simulink subsystem "Day1_Scenario_1"  (R2024a)
settings: Solver=VariableStepAuto  StartTime=0.0  StopTime=10.0  RelTol=1e-3
libraries: CarMaker4SL x1
settings Model: Creator=junhyung.cha  LastModifiedBy=User

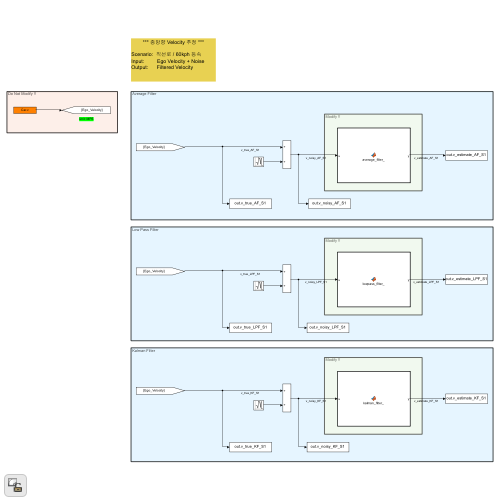
[thumbnail: Simulink's stored preview of the top-level diagram]
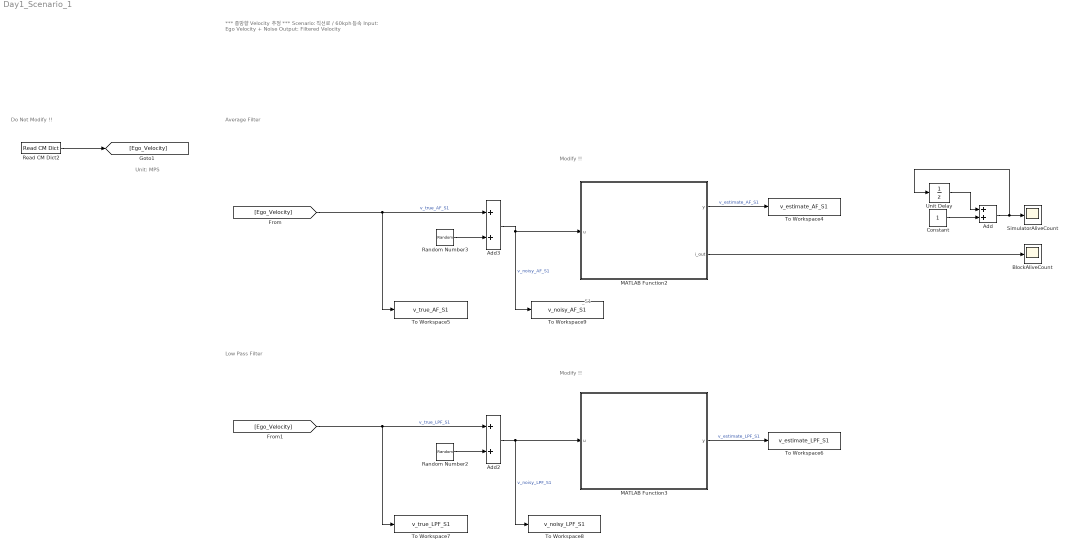
== system Day1_Scenario_1 ==
  note: _S1
  note: Modify !!
  note: Modify !!
  note: Average Filter
  note: Low Pass Filter
  note: *** 종방향 Velocity 추정 ***
      |
      | Scenario: 직선로 / 60kph 등속
      | Input: Ego Velocity + Noise
      | Output: Filtered Velocity
  note: Do Not Modify !!
  note: Unit: MPS
  Add : Sum
  Add2 : Sum
  Add3 : Sum
  BlockAliveCount : Scope
  Constant : Constant  SampleTime=-1
  MATLAB Function2 : MATLAB Function  TreatAsAtomicUnit=on
  MATLAB Function3 : MATLAB Function  TreatAsAtomicUnit=on
  Random Number2 : RandomNumber
  Random Number3 : RandomNumber
  Read CM Dict2 : CarMaker4SL/Read CM Dict  xname=Car.v  xsync=off  xstime=Inherited
  SimulatorAliveCount : Scope
  To Workspace4 : ToWorkspace  VariableName=v_estimate_AF_S1  SaveFormat=Timeseries  SampleTime=-1
  To Workspace5 : ToWorkspace  VariableName=v_true_AF_S1  SaveFormat=Timeseries  SampleTime=-1
  To Workspace6 : ToWorkspace  VariableName=v_estimate_LPF_S1  SaveFormat=Timeseries  SampleTime=-1
  To Workspace7 : ToWorkspace  VariableName=v_true_LPF_S1  SaveFormat=Timeseries  SampleTime=-1
  To Workspace8 : ToWorkspace  VariableName=v_noisy_LPF_S1  SaveFormat=Timeseries  SampleTime=-1
  To Workspace9 : ToWorkspace  VariableName=v_noisy_AF_S1  SaveFormat=Timeseries  SampleTime=-1
  Unit Delay : UnitDelay  SampleTime=-1  HasFrameUpgradeWarning=on
  wires:
  Random Number2/1 -> Add2/2
  [Ego_Velocity] -> Add2/1, To Workspace7/1  "v_true_LPF_S1"
  Add2/1 -> MATLAB Function3/1(u), To Workspace8/1  "v_noisy_LPF_S1"
  MATLAB Function3/1(y) -> To Workspace6/1  "v_estimate_LPF_S1"
  MATLAB Function2/1(y) -> To Workspace4/1  "v_estimate_AF_S1"
  Random Number3/1 -> Add3/2
  [Ego_Velocity] -> Add3/1, To Workspace5/1  "v_true_AF_S1"
  Add3/1 -> MATLAB Function2/1(u), To Workspace9/1  "v_noisy_AF_S1"
  Read CM Dict2/1 -> [Ego_Velocity]
  Constant/1 -> Add/2
  Unit Delay/1 -> Add/1
  Add/1 -> SimulatorAliveCount/1, Unit Delay/1
  MATLAB Function2/2(i_out) -> BlockAliveCount/1

== matlab function Day1_Scenario_1/MATLAB Function3 ==
  settings: updateMethod=DISCRETE  sampleTime=0.05
  data: u input; y output
function y = lowpass_filter_(u)
    persistent y_prev alpha
    if isempty(y_prev)
        alpha = 0.95;
        y_prev = u;
    end
    y = alpha * y_prev + (1 - alpha) * u;
    y_prev = y;
end

== matlab function Day1_Scenario_1/MATLAB Function2 ==
  settings: updateMethod=DISCRETE  sampleTime=0.05
  data: u input; y output; i_out output
function [y,i_out] = average_filter_(u)

  persistent i prev_avg
  if isempty(i)
      i = 0;
      prev_avg = 0;
  end

  i = i + 1;
  i_out = i;

  y = prev_avg + (u - prev_avg) / i;
  prev_avg = y;

  end
